simulink model "Engine_Cooling_Fan_Control"  (R2025a)
settings: Solver=VariableStepAuto  StartTime=0.0  StopTime=30  RelTol=1e-3
libraries: simulink x2, SignalEditorBlockLib x1
settings Model: Creator=Rudransh  LastModifiedBy=Rudransh

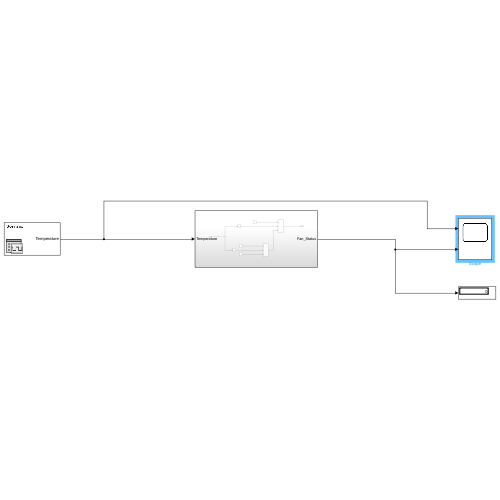
[thumbnail: Simulink's stored preview of the top-level diagram]
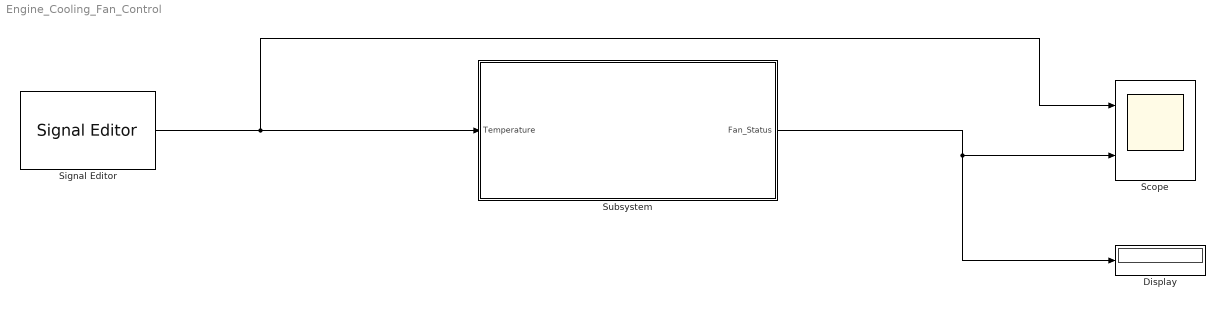
== system Engine_Cooling_Fan_Control ==
  Display : Display
  Scope : Scope  NumInputPorts=2
      settings: Title=FanStatus  ActiveDisplayYMinimum=0  ActiveDisplayYMaximum=2
  Signal Editor : SignalEditorBlockLib/Signal Editor  FileName=C:\Projects_ESD\AUTOSAR_CARSYSTEM\Engine_Cooling_Fan_Control\Scenario\Scenario5.mat  ActiveScenario=Scenario  ActiveSignal=Temperature  IsBus=off  OutputBusObjectStr=Bus: BusObject  SampleTime=0  ZeroCross=off  OutputAfterFinalValue=Setting to zero  Unit=inherit  PreserveSignalName=on  ApplySigPropsToAllScenarios=on  ApplySigPropsToAllSignals=off  SignalPropertySource=Dialog parameters
  Subsystem : Subsystem
  wires:
  Subsystem/1(Fan_Status) -> Display/1, Scope/2
  Signal Editor/1 -> Scope/1, Subsystem/1(Temperature)

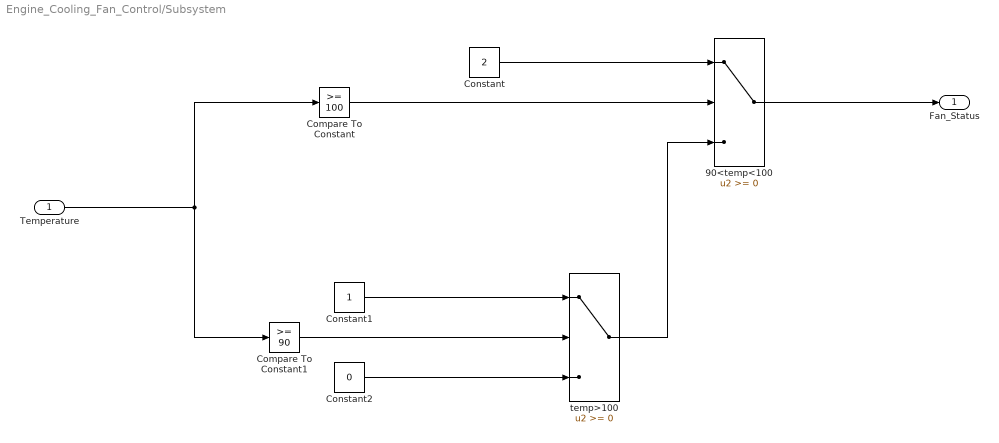
== system Engine_Cooling_Fan_Control/Subsystem ==
  Temperature : Inport
  90<temp<100 : Switch  SaturateOnIntegerOverflow=off  InputSameDT=off
  Compare To Constant : simulink/Logic and Bit Operations/Compare To Constant  relop=>=  const=100  OutDataTypeStr=boolean
  Compare To Constant1 : simulink/Logic and Bit Operations/Compare To Constant  relop=>=  const=90  OutDataTypeStr=boolean
  Constant : Constant  Value=2
  Constant1 : Constant
  Constant2 : Constant  Value=0
  temp>100 : Switch  SaturateOnIntegerOverflow=off  InputSameDT=off
  Fan_Status : Outport
  wires:
  Constant1/1 -> temp>100/1
  Constant2/1 -> temp>100/3
  Compare To Constant/1 -> 90<temp<100/2
  temp>100/1 -> 90<temp<100/3
  Constant/1 -> 90<temp<100/1
  Temperature/1 -> Compare To Constant1/1, Compare To Constant/1
  90<temp<100/1 -> Fan_Status/1
  Compare To Constant1/1 -> temp>100/2
